simulink model "sim_2D_underactuated"  (R2024b)
settings: Solver=FixedStepAuto  StartTime=0.0  StopTime=50  FixedStep=0.0001  RelTol=1e-3
settings Model: Creator=olive  LastModifiedBy=olivermcnaughton
settings DebuggingCC: UnderSpecifiedDimensionMsg=warning

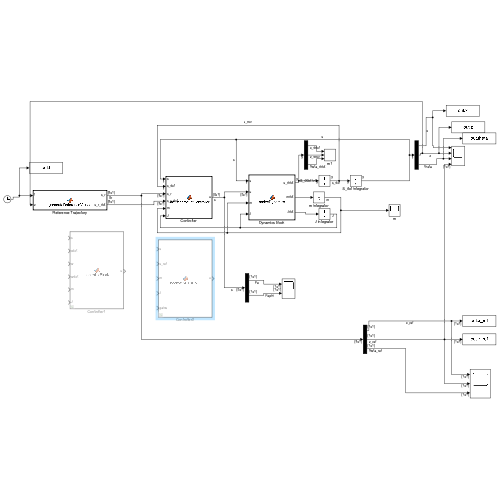
[thumbnail: Simulink's stored preview of the top-level diagram]
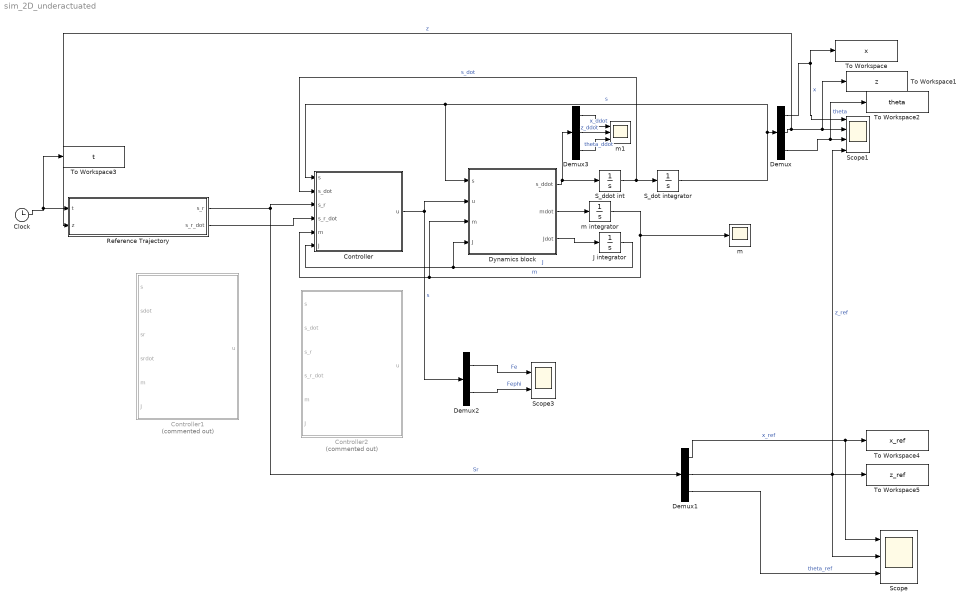
== system sim_2D_underactuated ==
  Clock : Clock
  Controller : MATLAB Function  TreatAsAtomicUnit=on
  Controller1 : MATLAB Function  Commented=on  TreatAsAtomicUnit=on
  Controller2 : MATLAB Function  Commented=on  TreatAsAtomicUnit=on
  Demux : Demux  Outputs=3
  Demux1 : Demux  Outputs=3
  Demux2 : Demux  Outputs=2
  Demux3 : Demux  Outputs=3
  Dynamics block : MATLAB Function  TreatAsAtomicUnit=on
  J integrator : Integrator  InitialCondition=5
  Reference Trajectory : MATLAB Function  TreatAsAtomicUnit=on
  S_ddot int : Integrator  InitialCondition=[0; 0; 0]
  S_dot integrator : Integrator  InitialCondition=[0.3;1;0]
  Scope : Scope  NumInputPorts=3
  Scope1 : Scope  NumInputPorts=4
  Scope3 : Scope  NumInputPorts=2
  To Workspace : ToWorkspace  VariableName=x  SaveFormat=Timeseries  SampleTime=-1
  To Workspace1 : ToWorkspace  VariableName=z  SaveFormat=Timeseries  SampleTime=-1
  To Workspace2 : ToWorkspace  VariableName=theta  SaveFormat=Timeseries  SampleTime=-1
  To Workspace3 : ToWorkspace  VariableName=t  SaveFormat=Timeseries  SampleTime=-1
  To Workspace4 : ToWorkspace  VariableName=x_ref  SaveFormat=Timeseries  SampleTime=-1
  To Workspace5 : ToWorkspace  VariableName=z_ref  SaveFormat=Timeseries  SampleTime=-1
  m : Scope
  m integrator : Integrator  InitialCondition=25
  m1 : Scope  NumInputPorts=3
  wires:
  Dynamics block/1(s_ddot) -> Demux3/1, S_ddot int/1
  Dynamics block/2(mdot) -> m integrator/1
  Dynamics block/3(Jdot) -> J integrator/1
  S_ddot int/1 -> Controller/2(s_dot), S_dot integrator/1  "s_dot"
  S_dot integrator/1 -> Controller/1(s), Dynamics block/1(s), Demux/1  "s"
  J integrator/1 -> Dynamics block/4(J), Controller/6(J)  "J"
  m integrator/1 -> Dynamics block/3(m), Controller/5(m), m/1  "m"
  Demux/1 -> To Workspace/1, Scope1/1  "x"
  Demux/2 -> Reference Trajectory/2(z), To Workspace1/1, Scope1/2  "z"
  Demux/3 -> To Workspace2/1, Scope1/3  "theta"
  Demux2/2 -> Scope3/2  "Fephi"
  Demux2/1 -> Scope3/1  "Fe"
  Controller/1(u) -> Demux2/1, Dynamics block/2(u)  "s"
  Clock/1 -> To Workspace3/1, Reference Trajectory/1(t)
  Reference Trajectory/1(s_r) -> Demux1/1, Controller/3(s_r)  "Sr"
  Demux1/2 -> To Workspace5/1, Scope1/4, Scope/2  "z_ref"
  Demux1/1 -> Scope/1, To Workspace4/1  "x_ref"
  Demux1/3 -> Scope/3  "theta_ref"
  Reference Trajectory/2(s_r_dot) -> Controller/4(s_r_dot)
  Demux3/1 -> m1/1  "x_ddot"
  Demux3/2 -> m1/2  "z_ddot"
  Demux3/3 -> m1/3  "theta_ddot"

== matlab function sim_2D_underactuated/Reference Trajectory ==
  data: s_r output; s_r_dot output; t input; z input
function [s_r, s_r_dot] = generateReferenceValues(t,z)
% Generates constant reference position and velocity values for x, z, and theta
% Outputs:
%   sr: Reference position vector [x_ref; z_ref; theta_ref]
%   srdot: Reference velocity vector [x_dot_ref; z_dot_ref; theta_dot_ref]

%set position and time for each segment
%set to 1 for a hover, set 0 otherwise
hover = 0;
%set to 1 for a falcon 9 style boost back burn, set 0 otherwise
falcon_9_traj=1;
%set to 1 if tuning
if hover ==1
    x_ref = 0;
    z_ref = 1;
    theta_ref = 0;

    x_dot_ref = 0;
    z_dot_ref = 0;
    theta_dot_ref = 0;

    x_ddot_ref = 0;
    z_ddot_ref = 0;
    theta_ddot_ref = 0;
end

if falcon_9_traj ==1
    %the rocket follows a trajectory of a half sine wave (middle part) then a
    %semi circle for the top of the boostback portion 
    %then a straight line downwards
    %End time of half sinewave
    T1 = 10;
    %End point of half sine wave
    x1 = 30;
    z1 = 40;
    
    %End time of semi circle 
    T2 = 20;
    %End point of semi circle
    x2 = 15; %gives you the position of the other side of the semi circle
    z2 = 40; %this should equal z1
    
    %Landing time of rocket
    T3 = 50;
    %Landing point of rocket
    x3 = 20; % this should be equal to x2
    z3 = 0;
    
    % Initialize reference values for safety
    x_ref = 0;
    z_ref = 0;
    theta_ref = 0;

    x_dot_ref = 0;
    z_dot_ref = 0;
    theta_dot_ref = 0;

    x_ddot_ref = 0;
    z_ddot_ref = 0;
    theta_ddot_ref = 0;

    %The first half sine wave
    if t<T1
        %reference positions
        x_ref = (-sin((pi/2) + pi*t/T1)+1)*x1/2;
        z_ref = z1*t/T1;
        theta_ref = atan(sin(pi*t/T1));
        
        %Reference Velocities
        x_dot_ref = (-pi/T1)*cos((pi/2) + pi*t/T1)*x1/2;
        z_dot_ref = z1/T1;
        theta_dot_ref = (pi/T1)*cos(pi*t/T1)/(sin(pi*t/T1)^2 + 1);

        %Reference Accelerations
        x_ddot_ref = ((pi/T1)^2)*sin((pi/2) + pi*t/T1)*x1/2;
        z_ddot_ref = 0;
        k = pi/T1;
        theta_ddot_ref = -k^2 * sin(k * t) * (3 - sin(k * t)^2) / (1 + sin(k * t)^2)^2;
    end
    %now doing the semi circle
    if t<T2 && t>=T1
        %calculate radius
        r = (x1-x2)/2; %radius 
        h = (x1+x2)/2; %x position for centre of circle
        dT = T2-T1; %Time between points
        dX = x1-x2;
        thetaMax = pi/4; %max angle at when halfway through the semi circle 
        teff = t -T1; %need to "zero" compared to the RHS of the semi circle
        %reference positions
        x_ref = h + r*cos(pi*teff/dT);
        z_ref = z1 + r*sin(pi*teff/dT);
        theta_ref = thetaMax*sin(2*pi*teff/dT + pi);
        %Reference Velocities
        x_dot_ref = (-pi/dT)*r*sin(pi*teff/dT);
        z_dot_ref = (pi/dT)*r*cos(pi*teff/dT);
        theta_dot_ref = thetaMax*(2*pi/dT)*cos(2*pi*teff/dT + pi);

        %Reference Accelerations
        x_ddot_ref = -(pi^2/dT^2)*r*cos(pi*teff/dT);
        z_ddot_ref = -(pi^2/dT^2)*r*sin(pi*teff/dT);
        theta_ddot_ref = -4*(pi^2/dT^2)*thetaMax*sin(pi*teff/dT + pi);
    end
    %now it is landing
    if t>=T2 
        % Position
        x_ref = x2; % Assuming no horizontal movement during landing
        z_ref = z2-4*(t-T2);
        theta_ref = 0; % No rotation during landing
        
        % Velocity
        x_dot_ref = 0;
        if z<5
            z_dot_ref = 0;
            z_ref = 0;
        else 
            z_dot_ref = -4;
        end
        
        theta_dot_ref = 0;
        
        % Acceleration
        x_ddot_ref = 0;
        z_ddot_ref = 0;
        theta_ddot_ref = 0;
    end
    if t>T3
        x_ref = x2;
        z_ref = 0;
        theta_ref = 0; % No rotation during landing
    end
    
end
% Output reference values
s_r = [x_ref; z_ref; theta_ref];
s_r_dot = [x_dot_ref; z_dot_ref; theta_dot_ref];
s_r_ddot = [x_ddot_ref; z_ddot_ref; theta_ddot_ref];
end

== matlab function sim_2D_underactuated/Dynamics block ==
  data: s input size=3; u input; m input; J input; s_ddot output size=3; mdot output size=1; Jdot output size=1
function [s_ddot,mdot,Jdot] = rocketDynamics(s,u,m,J)

%initialise states
L = 1;
alpha1 = 0.009;
alpha2 = 0.005;
beta = 0.03;
g = 9.81;

%extract states
Fe = u(1);
phi = u(2);

theta = s(3);

%find mdot and Jdot
mdot = -alpha1*(beta*Fe);
Jdot = -alpha2*(beta*Fe);
%update mdot and Jdot

x_ddot = Fe*(theta + phi)/m;
z_ddot = -g + Fe*(1-theta*phi)/m; 
theta_ddot = Fe*phi*L/J;

s_ddot = [x_ddot;z_ddot;theta_ddot];

end

== matlab function sim_2D_underactuated/Controller1 ==
  data: s input; sdot input; sr input; srdot input; m input; J input; u output
function u  = controllerBlock(s,sdot,sr,srdot,m,J)
% controllerBlock computes control input u for a 3-DOF system.
%
% Inputs:
%   s       = [x; z; theta] (actual position/orientation)
%   sr      = [x_r; z_r; theta_r] (reference)
%   sdot    = [xdot; zdot; thetadot] (actual velocity)
%   srdot   = [x_rdot; z_rdot; theta_rdot] (reference velocity)
%   sddot   = [xddot; zddot; thetaddot] (actual acceleration)
%   srddot  = [x_rddot; z_rddot; theta_rddot] (reference acceleration)
%
% Output:
%   u       = control input 
    %initialise states
    L1 = 1;
    Ln = 1;
    g = 9.81;


    % == Extract actual states ==
    x       = s(1); 
    z       = s(2);
    theta   = s(3);
    
    % == Extract reference states ==
    xr      = sr(1);
    zr      = sr(2);
    thetar  = sr(3);

    % == Extract actual velocities ==
    xdot    = sdot(1);
    zdot    = sdot(2);
    thetadot= sdot(3);

    % == Extract reference velocities ==
    xrdot   = srdot(1);
    zrdot   = srdot(2);
    thetardot = srdot(3);
    
    % System dynamics
    fs = [0;-g;0];
    gs = [theta/m 1/m; 1/m -theta/m; 0 -(L1+Ln)/J]; 

    % == Errors ==
    % Position error:
    e  = [x - xr; z - zr; theta - thetar];
    
    % Velocity error:
    e_dot  = [xdot - xrdot; zdot - zrdot; thetadot - thetardot]; 

    % Sliding Mode Control Parameters
    lambda = 5;   % Tuning parameter for speed of convergence
    k = 10;       % Gain to ensure sliding condition

    %compute the sliding surface
    S = e_dot + lambda * e;
    
    % Compute SMC Control Input
    u = -pinv(gs) * (fs + lambda * e_dot + k * sign(S));
    
    %set bounds for u 
    u(1) =  max(0, min(6486, u(1)));  %We need to bound Fe min = 0N max = 6486N
    u(2) =  max(-1678.7, min(1678.7, u(2)));  %Need to Bound Fephi

== matlab function sim_2D_underactuated/Controller ==
  data: s input; s_dot input; s_r input; s_r_dot input; m input; J input; u output
function u = BacksteprocketController(s, s_dot, s_r, s_r_dot, m, J)
% rocketController - Backstepping-based controller for rocket dynamics
%
% Inputs:
%   s     - Current state vector [x; z; theta; x_dot; z_dot; theta_dot]
%   s_ref - Reference state vector [x_ref; z_ref; x_dot_ref; z_dot_ref; x_ddot_ref; z_ddot_ref]
%   m     - Current mass of the rocket
%   J     - Current moment of inertia
%   gains - Struct containing control gains (k1, k2, k3, k4)
%
% Output:
%   u     - Control input vector [Fe; phi]

% Extract current states
x = s(1);
z = s(2);
theta = s(3);
x_dot = s_dot(1);
z_dot = s_dot(2);
theta_dot = s_dot(3);

% Extract reference states
x_ref = s_r(1);
z_ref = s_r(2);
x_dot_ref = s_r(3);
z_dot_ref = s_r_dot(1);
x_ddot_ref = s_r_dot(2);
z_ddot_ref = s_r_dot(3);

% Control gains
k1 = 1.5;
k2 = 2.2;
k3 = 3;
k4 = 4;

% Step 1: Compute errors
e1 = x - x_ref;
e2 = z - z_ref;

% Virtual control laws (Backstepping)
alpha1 = x_dot_ref - k1 * e1;
alpha2 = z_dot_ref - k3 * e2;

z1 = x_dot - alpha1;
z2 = z_dot - alpha2;

% Compute virtual inputs
v1 = x_ddot_ref - k1 * (x_dot - x_dot_ref) - k2 * z1;
v2 = z_ddot_ref - k3 * (z_dot - z_dot_ref) - k4 * z2;

% Recover actual control inputs (Fe and phi)
g = 9.81; % Gravity

denominator = v1 * theta + (v2 + g);

% Avoid division by zero
if abs(denominator) < 1e-6
    denominator = sign(denominator) * 1e-6;
end

phi = (v1 - (v2 + g) * theta) / denominator;
Fe = m * v1 / (theta + phi);

% Output control vector
u = [Fe; phi];

end

== matlab function sim_2D_underactuated/Controller2 ==
  data: s input; s_dot input; s_r input; s_r_dot input; m input; J input; u output
function u = backstepPlusSMC(s, s_dot, s_r, s_r_dot, m, J)
% rocketControllerSMC - Backstepping-based controller with Sliding Mode Control (SMC) for attitude
%
% Inputs:
%   s     - Current state vector [x; z; theta; x_dot; z_dot; theta_dot]
%   s_ref - Reference state vector [x_ref; z_ref; x_dot_ref; z_dot_ref; x_ddot_ref; z_ddot_ref]
%   m     - Current mass of the rocket
%   J     - Current moment of inertia
%   gains - Struct containing control gains (k1, k2, k3, k4, lambda, eta)
%
% Output:
%   u     - Control input vector [Fe; phi]

% Extract current states
x = s(1);
z = s(2);
theta = s(3);
x_dot = s_dot(4);
z_dot = s_dot(5);
theta_dot = s_dot(6);

% Extract reference states
x_ref = s_r(1);
z_ref = s_r(2);
x_dot_ref = s_r(3);
z_dot_ref = s_r_dot(4);
x_ddot_ref = s_r_dot(5);
z_ddot_ref = s_r_dot(6);

% Control gains
k1 = gains.k1;
k2 = gains.k2;
k3 = gains.k3;
k4 = gains.k4;

% SMC gains for attitude control
lambda = gains.lambda;  % Sliding surface gain
eta = gains.eta;        % Reaching law gain

% Constants
g = 9.81; % Gravity
L = 1;    % Lever arm (distance from center of mass to thrust vector)

%% Outer Loop - Position Control (Backstepping)
% Position errors
e1 = x - x_ref;
e2 = z - z_ref;

% Virtual control laws (Backstepping)
alpha1 = x_dot_ref - k1 * e1;
alpha2 = z_dot_ref - k3 * e2;

% Backstepping errors
z1 = x_dot - alpha1;
z2 = z_dot - alpha2;

% Virtual inputs (desired accelerations)
v1 = x_ddot_ref - k1 * (x_dot - x_dot_ref) - k2 * z1;
v2 = z_ddot_ref - k3 * (z_dot - z_dot_ref) - k4 * z2;

%% Desired Orientation from Outer Loop
theta_des = atan2(v1, v2 + g); % Desired pitch angle to achieve (v1, v2)

%% Inner Loop - Sliding Mode Control for Attitude
% Sliding surface
s_theta = theta_dot + lambda * (theta - theta_des);

% SMC control law (reaching law)
torque = -lambda * theta_dot - eta * sign(s_theta); % Torque command to stabilize theta

%% Recover Actual Control Inputs (Fe and phi)
% Total thrust magnitude
Fe = m * sqrt(v1^2 + (v2 + g)^2); 

% Thrust vector angle phi based on required torque
% Using: torque = Fe * L * sin(phi) => phi = asin(torque / (Fe * L))
phi = asin(torque / (Fe * L));

% Handle numerical issues when phi is close to limits
phi = max(min(phi, pi/4), -pi/4); % Limit phi within ±45 degrees

%% Output Control Vector
u = [Fe; phi];

end
